simulink model "generic_IVS"  (R2024a)
settings: Solver=FixedStepDiscrete  StartTime=0.0  StopTime=inf  FixedStep=0.001  RelTol=1e-3  EnableMultiTasking=on
undefined symbols (not defined in the file): filtered_route_waypoint_raw, route1_waypoint_x, route1_waypoint_y, route2_waypoint_raw, route2_waypoint_x, route2_waypoint_y, route3_waypoint_x, route3_waypoint_y, route4_waypoint_x, route4_waypoint_y, route5_waypoint_x, route5_waypoint_y
libraries: CarMaker4SL x125, slpidlib x7, simulink x1, robotalgslib x1
(part 5 of 5)

== matlab function generic_IVS/CarMaker/Subsystem/Final Project/Scenario 1/Triggered Subsystem2/Function-Call Subsystem/MATLAB Function4 ==
  data: start input; goal input; obstacle_list input; full_path output
function full_path = main_rrt_rs(start, goal, obstacle_list) %#codegen
    disp("MAP making start")
    space = [5.5, 47.5, -44.9, -4.1];
    max_iter = 15000; step_size = 0.4; goal_sample_rate = 0.6; radius = 15;
    MAX_NODES = 5000;
    default_node = struct('pos', zeros(1,3), 'parent', int32(0), 'cost', Inf);
    nodes = repmat(default_node, 1, MAX_NODES);
    nodes(1).pos = start(:)';
    nodes(1).parent = int32(0);
    nodes(1).cost = 0.0;
    node_count = int32(1);
    goal = reshape(goal, 1, 3);
    start = reshape(start, 1, 3);

    c_best = inf; best_goal_node = int32(-1);

    for iter = 1:max_iter
        if rand < goal_sample_rate
            sample = goal;
        elseif isfinite(c_best)
            sample = informed_sample(start, goal, c_best, space);
        else
            sample = [ ...
                rand_range(space(1), space(2)), ...
                rand_range(space(3), space(4)), ...
                rand * 2 * pi ...
                ];
        end
        sample = reshape(sample, 1, 3);
        min_dist = inf;
        nearest_id = int32(1);
        for i = 1:node_count
            d = norm(nodes(i).pos(1:2) - sample(1:2));
            if d < min_dist
                min_dist = d;
                nearest_id = int32(i);
            end
        end
        nearest_node = nodes(nearest_id);

        theta = atan2(sample(2) - nearest_node.pos(2), sample(1) - nearest_node.pos(1));
        new_pos = [nearest_node.pos(1:2) + step_size * [cos(theta), sin(theta)], theta];

        if ~collision_check_line(nearest_node.pos, new_pos, obstacle_list, space)
            new_node = struct('pos', new_pos, ...
                'parent', int32(nearest_id), ...
                'cost', nearest_node.cost + norm(new_pos(1:2) - nearest_node.pos(1:2)));

            for i = 1:node_count
                if norm(nodes(i).pos(1:2) - new_node.pos(1:2)) < radius
                    temp_cost = nodes(i).cost + norm(nodes(i).pos(1:2) - new_node.pos(1:2));
                    if temp_cost < new_node.cost && ~collision_check_line(nodes(i).pos, new_node.pos, obstacle_list, space)
                        new_node.cost = temp_cost;
                        new_node.parent = int32(i);
                    end
                end
            end

            if node_count < MAX_NODES
                node_count = node_count + 1;
                nodes(node_count) = new_node;
            end

            if norm(new_node.pos(1:2) - goal(1:2)) < 10 && abs(wrapToPi(new_node.pos(3) - goal(3))) < deg2rad(360)
                if new_node.cost < c_best
                    c_best = new_node.cost;
                    best_goal_node = node_count;
                end
            end
        end
    end

    function yaw = wrapToPi(yaw)
        while yaw > pi
            yaw = yaw - 2*pi;
        end
        while yaw < -pi
            yaw = yaw + 2*pi;
        end
    end

    if best_goal_node > 0
        path_temp = zeros(300, 3);
        count = int32(0);
        current = best_goal_node;
        while current > 0
            count = count + 1;
            path_temp(count,:) = nodes(current).pos;
            current = nodes(current).parent;
        end
        rrt_path = flipud(path_temp(1:count,:));
        rrt_path = path_clothoid_smoothing(rrt_path);
        n_rrt = size(rrt_path, 1);

        full_path = NaN(300,3);
        full_path(1:n_rrt, :) = rrt_path;
        full_path(n_rrt + 1, :) = goal;  % ✅ goal을 마지막에 추가
    else
        full_path = NaN(300,3);
        disp('No Map Path!')
    end

    function r = rand_range(a, b) %#codegen
        r = a + (b - a) * rand;
    end

    disp("MAP function finish")
end
function sample = informed_sample(start, goal, c_max, space) %#codegen
    % === 고정된 출력: 반드시 [1×3] 벡터 ===
    sample = zeros(1, 3);

    % === 타원 파라미터 계산 ===
    c_min = norm(goal(1:2) - start(1:2));
    a = c_max / 2;
    b = sqrt(max(1e-6, c_max^2 - c_min^2)) / 2;
    theta = atan2(goal(2) - start(2), goal(1) - start(1));
    cos_t = cos(theta);
    sin_t = sin(theta);
    mid = 0.5 * (start(1:2) + goal(1:2));

    % === 고정 반복 횟수 시도 (예: 50회) ===
    for i = 1:50
        x = a * (2 * rand - 1);  % [-a, a]
        y = b * (2 * rand - 1);  % [-b, b]

        % 타원 내부 점만 사용
        if (x^2 / a^2 + y^2 / b^2) <= 1
            pos_x = cos_t * x - sin_t * y + mid(1);
            pos_y = sin_t * x + cos_t * y + mid(2);
            yaw   = 2 * pi * rand;

            sample(1) = pos_x;
            sample(2) = pos_y;
            sample(3) = yaw;
            return;
        end
    end

    % 실패 시 fallback: goal 반환
    sample = goal(:)';  % [1×3] 형태 유지
end

function smooth_path = path_clothoid_smoothing(path)
    if size(path, 1) < 3
        smooth_path = path;
        return;
    end

    fixed_points = false(size(path, 1), 1);
    for i = 2:size(path, 1) - 1
        prev = path(i - 1, 1:2);
        curr = path(i, 1:2);
        next = path(i + 1, 1:2);
        angle1 = atan2(curr(2) - prev(2), curr(1) - prev(1));
        angle2 = atan2(next(2) - curr(2), next(1) - curr(1));
        if abs(angle1 - angle2) < deg2rad(5)
            fixed_points(i) = true;
        end
    end

    x = path(:, 1); y = path(:, 2); yaw = path(:, 3);
    s = cumsum([0; sqrt(diff(x).^2 + diff(y).^2)]);
    ts = linspace(0, s(end), 5 * numel(s));
    x_smooth = interp1(s(~fixed_points), x(~fixed_points), ts, 'pchip', 'extrap');
    y_smooth = interp1(s(~fixed_points), y(~fixed_points), ts, 'pchip', 'extrap');
    yaw_unwrap = unwrap(yaw);
    yaw_smooth = interp1(s(~fixed_points), yaw_unwrap(~fixed_points), ts, 'pchip', 'extrap');

    dx = gradient(x_smooth); dy = gradient(y_smooth);
    ddx = gradient(dx); ddy = gradient(dy);
    curvature = abs((dx .* ddy - dy .* ddx) ./ (dx.^2 + dy.^2).^(3/2));
    max_curvature = 0.05;

    for k = 2:length(curvature)
        if curvature(k) > max_curvature
            factor = max_curvature / curvature(k);
            x_smooth(k) = x_smooth(k-1) + factor * (x_smooth(k) - x_smooth(k-1));
            y_smooth(k) = y_smooth(k-1) + factor * (y_smooth(k) - y_smooth(k-1));
        end
    end
    smooth_path = [x_smooth',...
                    y_smooth',...
                    wrapToPi(yaw_smooth')];
end





function is_collision = collision_check_line(start_pos, end_pos, obstacle_list, space) %#codegen
    % 간단한 선분-장애물 교차 검사: 샘플링 방식 사용
    n = 10;
    is_collision = false;
    for i = 0:n
        t = i / n;
        pos = (1 - t) * start_pos + t * end_pos;
        if collision_check_point(pos, obstacle_list, space)
            is_collision = true;
            return;
        end
    end
end

function is_collision = collision_check_point(pos, obstacle_list, space)
    x = pos(1); y = pos(2);
    if x < space(1) || x > space(2) || y < space(3) || y > space(4)
        is_collision = true;
        return;
    end
    is_collision = false;
    for i = 1:size(obstacle_list, 1)
        dx = x - obstacle_list(i,1);
        dy = y - obstacle_list(i,2);
        if hypot(dx, dy) < obstacle_list(i,3) + 1.5
            is_collision = true;
            return;
        end
    end
end

== matlab function generic_IVS/CarMaker/Subsystem/Final Project/Scenario 1/Tollgate/Get frenet1/MATLAB Function2 ==
  settings: sampleTime=0.05
  data: x input; y input; mapx input; mapy input; next_wp input; frenet_s output; frenet_d output; n_x output; n_y output
function [frenet_s, frenet_d,n_x, n_y] = get_frenet(x, y, mapx, mapy, next_wp)

% 예외 처리: 첫 번째 웨이포인트면 1로 고정
if next_wp == 1
    prev_wp = 1;
else
    prev_wp = next_wp - 1;
end

% 웨이포인트 벡터 (경로 벡터)
n_x = mapx(next_wp) - mapx(prev_wp);
n_y = mapy(next_wp) - mapy(prev_wp);
x_x = x - mapx(prev_wp);
x_y = y - mapy(prev_wp);

% 투영 계산 (단위가 아닌 비율)
proj_norm = (x_x * n_x + x_y * n_y) / (n_x^2 + n_y^2);
proj_x = proj_norm * n_x;
proj_y = proj_norm * n_y;

% Frenet d 계산 (측방 오차)
frenet_d = sqrt((x_x - proj_x)^2 + (x_y - proj_y)^2);

% 외적 계산 (왼쪽/오른쪽 판단)
ego_vec = [x - mapx(prev_wp); y - mapy(prev_wp); 0];
map_vec = [n_x; n_y; 0];
d_cross = cross(ego_vec, map_vec);

if d_cross(3) > 0
    frenet_d = -frenet_d;
end

% Frenet s 계산 (누적 거리)
frenet_s = 0;
for i = 1:(prev_wp - 1)
    dx = mapx(i+1) - mapx(i);
    dy = mapy(i+1) - mapy(i);
    frenet_s = frenet_s + sqrt(dx^2 + dy^2);
end

frenet_s = frenet_s + sqrt(proj_x^2 + proj_y^2);

== matlab function generic_IVS/CarMaker/Subsystem/Final Project/Scenario 1/Tollgate/Get frenet1/MATLAB Function3 ==
  data: route2_waypoint_raw input; map_x output; map_y output
function [map_x,map_y] = map(route2_waypoint_raw)

map_x = route2_waypoint_raw(:,1);
map_y = route2_waypoint_raw(:,2);

== matlab function generic_IVS/CarMaker/Subsystem/Final Project/Scenario 1/Tollgate/Get frenet1/MATLAB Function4 ==
  data: frenet_s_in input; frenet_s_out output
function frenet_s_out = safe_frenet_s(frenet_s_in)
% 입력:
%   s_in  : 현재 계산된 frenet_s
% 출력:
%   s_out : 점프가 제한된 frenet_s 출력

    % 이전 frenet_s 저장용 persistent 변수
    persistent prev_s
    if isempty(prev_s)
        prev_s = 0;
    end

    % 허용 가능한 최대 변화량 (단위: m)
    THRESHOLD = 900.0;

    % 변화량이 너무 크면 이전 값 유지
    if abs(frenet_s_in - prev_s) > THRESHOLD
        frenet_s_out = prev_s;
    else
        frenet_s_out = frenet_s_in;
        prev_s = frenet_s_in;
    end
end

== matlab function generic_IVS/CarMaker/Subsystem/Final Project/Scenario 1/Tollgate/ACC PD1 ==
  settings: sampleTime=0.05
  data: obs_s_array input; desired_ax output; ego_s input; error_min output; desired_ax_cruise input; ego_d input; d_array input
function [desired_ax, error_min] = longitudinal_space_pid_controller_traffic(obs_s_array, ego_s, desired_ax_cruise, ego_d, d_array)
% obs_s_array : 8×1 double (각 traffic 차량의 s 좌표)
% ego_s       : 자차량 s 좌표
% desired_ax  : 가속도 출력 (m/s^2)
% error_min   : 선택된 전방 차량과의 거리 오차
% ego_d       : 자차의 d 좌표 (자차와 각 traffic의 d 값 차이 비교)
% d_array     : 각 traffic 차량들의 d 좌표

    % === PID gain 설정 ===
    Kp = 0.17; %0.4, 0.2, 0.3
    Ki = 0;
    Kd = 0;

    % === 목표 간격 ===
    target_distance = 29;  %m
    % 30, 25, 30, 28

    % === 상태 유지용 변수 ===
    persistent integral_error prev_error
    if isempty(integral_error)
        integral_error = 0;
        prev_error = 0;
    end

    dt = 0.05;  % 샘플링 주기

    % === 전방 차량 필터링 ===
    delta_s = obs_s_array - ego_s;
    front_idx = find(delta_s > 0);

    if isempty(front_idx)
        % 전방 차량 없음 → 정상 주행 유지 (가속)
        desired_ax = desired_ax_cruise;
        error_min = NaN;
        return;
    end

    % === 가장 가까운 전방 차량 선택 및 d 차이 확인 ===
    target_idx = -1;
    for i = 1:length(front_idx)
        idx = front_idx(i);
        d_diff = abs(ego_d - d_array(idx)); % 자차와 각 traffic 차량 간의 d 차이

        if d_diff < 1.75
            target_idx = idx;
            break;  % d 차이가 1.75보다 작으면 해당 차량을 선택
        end
    end

    % d 차이가 1.75보다 작은 차량이 없다면 크루즈 유지
    if target_idx == -1
        desired_ax = desired_ax_cruise;
        error_min = NaN;
        return;
    end

    % === 선택된 차량의 s 값으로 거리 계산 ===
    min_dist = delta_s(target_idx);
    % error_min 계산: 선택된 전방 차량과 자차 간의 거리 차이
    error_min = min_dist - target_distance;

    % === PID 계산 ===
    integral_error = integral_error + error_min * dt;
    derivative_error = (error_min - prev_error) / dt;

    % === s 거리 계산 후 ACC 작동 여부 ===
    if min_dist > target_distance
        % 전방 차량과의 거리가 목표 거리보다 크면 cruise 유지
        desired_ax = desired_ax_cruise;
    else
        % 그렇지 않으면 PID로 가속도 조절
        desired_ax = Kp * error_min + Ki * integral_error + Kd * derivative_error;
    end

    % === 상태 업데이트 ===
    prev_error = error_min;
end

%%
% function [desired_ax, error_min] = longitudinal_space_pid_controller_traffic(obs_s_array, ego_s, desired_ax_cruise, ego_d, d_array)
% % obs_s_array : 8×1 double (각 traffic 차량의 s 좌표)
% % ego_s       : 자차량 s 좌표
% % desired_ax  : 가속도 출력 (m/s^2)
% % error_min   : 선택된 전방 차량과의 거리 오차
% % ego_d       : 자차의 d 좌표 (자차와 각 traffic의 d 값 차이 비교)
% % d_array     : 각 traffic 차량들의 d 좌표
% 
%     % === PID gain 설정 ===
%     Kp = 1.2;%1.6;
%     Ki = 0.1;%0.1;
%     Kd = 0.038;%0.3;
% 
%     % === 목표 간격 ===
%     target_distance = 20;  % m
% 
%     % === 상태 유지용 변수 ===
%     persistent integral_error prev_error
%     if isempty(integral_error)
%         integral_error = 0;
%         prev_error = 0;
%     end
% 
%     dt = 0.001;  % 샘플링 주기
% 
%     % === 전방 차량 필터링 ===
%     delta_s = obs_s_array - ego_s;
%     front_idx = find(delta_s > 0);
% 
%     if isempty(front_idx)
%         % 전방 차량 없음 → 정상 주행 유지 (가속)
%         desired_ax = desired_ax_cruise;
%         error_min = NaN;
%         return;
%     end
% 
%     % === 가장 가까운 전방 차량 선택 및 d 차이 확인 ===
%     target_idx = -1;
%     for i = 1:length(front_idx)
%         idx = front_idx(i);
%         d_diff = abs(ego_d - d_array(idx)); % 자차와 각 traffic 차량 간의 d 차이
% 
%         if d_diff < 1.75
%             target_idx = idx;
%             break;  % d 차이가 1.75보다 작으면 해당 차량을 선택
%         end
%     end
% 
%     % d 차이가 1.75보다 작은 차량이 없다면 크루즈 유지
%     if target_idx == -1
%         desired_ax = desired_ax_cruise;
%         error_min = NaN;
%         return;
%     end
% 
%     % === 선택된 차량의 s 값으로 거리 계산 ===
%     min_dist = delta_s(target_idx);
%     % error_min 계산: 선택된 전방 차량과 자차 간의 거리 차이
%     error_min = min_dist - target_distance;
% 
%     % === PID 계산 ===
%     integral_error = integral_error + error_min * dt;
%     derivative_error = (error_min - prev_error) / dt;
% 
%     % === s 거리 계산 후 ACC 작동 여부 ===
%     if min_dist > target_distance +30
%         % 전방 차량과의 거리가 목표 거리보다 크면 cruise 유지
%         desired_ax = desired_ax_cruise;
%     else
%         % 그렇지 않으면 PID로 가속도 조절
%         desired_ax = Kp * error_min + Ki * integral_error + Kd * derivative_error;
%     end
% 
%     % === 상태 업데이트 ===
%     prev_error = error_min;
% end

== matlab function generic_IVS/CarMaker/Subsystem/Final Project/Scenario 1/Drive/MATLAB Function1 ==
  settings: sampleTime=0.1
  data: x input; x_best output; y input; v input; map_x input; map_y input; obs_x input; obs_y input; y_best output; x_all output; y_all output; obs_Vx input; obs_Vy input; obs_ax input; obs_ay input; predicted_traj_x output; predicted_traj_y output; front_obstacle_flag output; road_curvature output

function [x_best, y_best, x_all, y_all, predicted_traj_x, predicted_traj_y, front_obstacle_flag, road_curvature] = ...
    FrenetTrajectoryGenerator(x, y, v, map_x, map_y, ...
    obs_x, obs_y, obs_Vx, obs_Vy, obs_ax, obs_ay)

% === 설정 ===
DF_set = [-3.5, 0, 3.5];  
K_J = 0.1; K_T = 0.1; K_D = 10.0; K_V = 1.0;
K_LAT = 2.0; K_LON = 1.0; K_SAFE_DIST = 100.0;

target_speed = 15;
T = 1.2; dt = 0.05;
ego_radius = 1.5;
LANE_WIDTH = 3.5;

M = length(DF_set);
N = round(T / dt);

x_all = zeros(N, M);
y_all = zeros(N, M);

obs_r = 2.0;
num_obs = length(obs_x);

% === 기준 경로 길이 계산 ===
map_s = zeros(length(map_x), 1);
for i = 2:length(map_x)
    dx = map_x(i) - map_x(i-1);
    dy = map_y(i) - map_y(i-1);
    map_s(i) = map_s(i-1) + hypot(dx, dy);
end

% === Ego 차량 위치 변환 ===
[s0, d0] = getFrenet(x, y, map_x, map_y, map_s);
si = s0; si_d = v; si_dd = 0;
di = d0; di_d = 0; di_dd = 0;

% === 주변 차량 Frenet 기반 예측 정보 ===
pred_vehicles = zeros(num_obs, 3);  % [s0, v0, a0]
pred_d0 = zeros(num_obs, 1);        % 초기 lateral offset
predicted_traj_x = zeros(N, num_obs);
predicted_traj_y = zeros(N, num_obs);

for j = 1:num_obs
    [s_obs, d_obs] = getFrenet(obs_x(j), obs_y(j), map_x, map_y, map_s);
    pred_d0(j) = d_obs;

    idx = find(map_s > s_obs,1)-1;
    idx = max(min(idx,length(map_x)-1),1);
    dx = map_x(idx+1)-map_x(idx);
    dy = map_y(idx+1)-map_y(idx);
    heading = atan2(dy,dx);

    vx = obs_Vx(j); vy = obs_Vy(j);
    ax = obs_ax(j); ay = obs_ay(j);

    v0 = vx*cos(heading) + vy*sin(heading);
    a0 = ax*cos(heading) + ay*sin(heading);

    pred_vehicles(j,:) = [s_obs, v0, a0];

    for i = 1:N
        t = (i-1)*dt;
        s_pred = s_obs + v0*t + 0.5*a0*t^2;
        d_pred = d_obs;
        [x_pred, y_pred] = getCartesian(s_pred, d_pred, map_x, map_y, map_s);
        predicted_traj_x(i,j) = x_pred;
        predicted_traj_y(i,j) = y_pred;
    end
end

% === Trajectory 후보 생성 및 평가 ===
costs = inf(1, M);
trajectories = cell(M,2);

for k = 1:M
    d_target = DF_set(k);

    % Lateral (Quintic)
    a0 = di; a1 = di_d; a2 = 0.5 * di_dd;
    A_lat = [T^3 T^4 T^5; 3*T^2 4*T^3 5*T^4; 6*T 12*T^2 20*T^3];
    b_lat = [d_target - a0 - a1*T - a2*T^2; -a1 - 2*a2*T; -2*a2];
    coeff_d = A_lat \ b_lat;

    % Longitudinal (Quartic)
    b0 = si; b1 = si_d; b2 = 0.5 * si_dd;
    A_lon = [3*T^2 4*T^3; 6*T 12*T^2];
    b_lon = [target_speed - b1 - 2*b2*T; -2*b2];
    coeff_s = A_lon \ b_lon;

    s_traj = zeros(N,1); d_traj = zeros(N,1);
    x_traj = zeros(N,1); y_traj = zeros(N,1);
    jerk_d = 0; jerk_s = 0;
    is_collision = false;
    min_gap = inf;

    for i = 1:N
        t = (i-1)*dt;
        s_t = b0 + b1*t + b2*t^2 + coeff_s(1)*t^3 + coeff_s(2)*t^4;
        d_t = a0 + a1*t + a2*t^2 + coeff_d(1)*t^3 + coeff_d(2)*t^4 + coeff_d(3)*t^5;

        s_traj(i) = s_t; d_traj(i) = d_t;

        j_d = 6*coeff_d(1) + 24*coeff_d(2)*t + 60*coeff_d(3)*t^2;
        j_s = 6*coeff_s(1) + 24*coeff_s(2)*t;
        jerk_d = jerk_d + j_d^2;
        jerk_s = jerk_s + j_s^2;

        [xg, yg] = getCartesian(s_t, d_t, map_x, map_y, map_s);
        x_traj(i) = xg;
        y_traj(i) = yg;

        % 정적 장애물: 같은 차선일 때만 판단
        for j = 1:num_obs
            [~, d_obs_static] = getFrenet(obs_x(j), obs_y(j), map_x, map_y, map_s);
            if abs(d_obs_static - d_t) < LANE_WIDTH / 2
                dist = hypot(xg - obs_x(j), yg - obs_y(j));
                if dist < (ego_radius + obs_r)
                    is_collision = true;
                end
            end
        end

        % 동적 장애물: 같은 차선만 판단
        for j = 1:num_obs
            s_pred = pred_vehicles(j,1) + pred_vehicles(j,2)*t + 0.5*pred_vehicles(j,3)*t^2;
            d_pred = pred_d0(j);
            ds = s_pred - s_t;
            dd = d_pred - d_t;
            dist_frenet = sqrt(ds^2 + dd^2);

            if abs(dd) < LANE_WIDTH / 2
                if dist_frenet < (ego_radius + obs_r)
                    is_collision = true;
                end
                if ds >= 0
                    min_gap = min(min_gap, ds);
                end
            end
        end
    end

    x_all(:,k) = x_traj;
    y_all(:,k) = y_traj;

    if ~is_collision
        d_diff = (d_traj(end))^2;
        v_diff = (target_speed - (s_traj(end)-s_traj(1))/T)^2;
        cost_lat = K_J*jerk_d + K_T*T + K_D*d_diff;
        cost_lon = K_J*jerk_s + K_T*T + K_V*v_diff;
        safe_cost = 0;
        if min_gap < 15
            safe_cost = K_SAFE_DIST * (15 - min_gap)^2;
        end
        costs(k) = K_LAT*cost_lat + K_LON*(cost_lon + safe_cost);
    end

    trajectories{k,1} = x_traj;
    trajectories{k,2} = y_traj;
end

% === 최적 trajectory 선택 ===
persistent prev_best_idx hold_count
if isempty(prev_best_idx)
    prev_best_idx = 2;
    hold_count = 0;
end

[best_cost, new_best_idx] = min(costs);
threshold = 5.0;
hold_limit = 3.0 / dt;
current_cost = costs(prev_best_idx);

if (new_best_idx ~= prev_best_idx) && ...
        (best_cost + threshold < current_cost || hold_count >= hold_limit)
    prev_best_idx = new_best_idx;
    hold_count = 0;
else
    new_best_idx = prev_best_idx;
    hold_count = hold_count + 1;
end

x_best = trajectories{new_best_idx,1};
y_best = trajectories{new_best_idx,2};

% === 전방 장애물 플래그 ===
front_obstacle_flag = 0;
SAFE_DETECT_DIST = 40;
for j = 1:num_obs
    s_pred = pred_vehicles(j,1);
    d_pred = pred_d0(j);
    ds = s_pred - s0;
    dd = d_pred - d0;
    if ds > 0 && ds < SAFE_DETECT_DIST && abs(dd) < LANE_WIDTH / 2
        front_obstacle_flag = 13;
        break;
    end
end

% === 전방 곡률 계산 ===
road_curvature = 0;
num_curv_pts = 10;
idx = find(map_s > s0, 1);
idx = idx(1);
if ~isempty(idx) && (idx + num_curv_pts <= length(map_s))
    xs = map_x(idx:idx+num_curv_pts);
    ys = map_y(idx:idx+num_curv_pts);
    dx = gradient(xs);
    dy = gradient(ys);
    ddx = gradient(dx);
    ddy = gradient(dy);
    kappa = abs(dx .* ddy - dy .* ddx) ./ (dx.^2 + dy.^2).^(3/2);
    kappa(~isfinite(kappa)) = 0;
    road_curvature = mean(kappa);
end

end



%% === 보조 함수 ===

function [s, d] = getFrenet(x, y, mapx, mapy, maps)
min_dist = inf; idx = 1;
for i = 1:length(mapx)-1
    dist = hypot(x - mapx(i), y - mapy(i));
    if dist < min_dist
        min_dist = dist;
        idx = i;
    end
end
dx = mapx(idx+1) - mapx(idx);
dy = mapy(idx+1) - mapy(idx);
seg_len = hypot(dx, dy);
proj = ((x - mapx(idx)) * dx + (y - mapy(idx)) * dy) / seg_len^2;
proj_x = mapx(idx) + proj * dx;
proj_y = mapy(idx) + proj * dy;
d = (x - proj_x) * (-dy/seg_len) + (y - proj_y) * (dx/seg_len);
s = maps(idx) + proj * seg_len;
end

function [x, y] = getCartesian(s, d, mapx, mapy, maps)
if s >= maps(end)
    s = maps(end) - 0.001;
end
idx_array = find(maps > s, 1);
if isempty(idx_array)
    idx = length(maps) - 1;
else
    idx = idx_array - 1;
end
if idx < 1
    idx = 1;
elseif idx >= length(mapx)
    idx = length(mapx) - 1;
end
mx0 = mapx(idx); mx1 = mapx(idx+1);
my0 = mapy(idx); my1 = mapy(idx+1);
dx_val = mx1 - mx0;
dy_val = my1 - my0;
heading = atan2(dy_val, dx_val);
ds = s - maps(idx);
base_x = mx0 + ds * cos(heading);
base_y = my0 + ds * sin(heading);
x = base_x - d * sin(heading);
y = base_y + d * cos(heading);
end

== matlab function generic_IVS/CarMaker/Subsystem/Final Project/Scenario 1/Drive/MATLAB Function4  ==
  settings: updateMethod=DISCRETE
  data: waypoint_x input; waypoint_y input; local_waypoints_ output; vehicle_position input; head input
function local_waypoints_ = global_to_local_waypoints(waypoint_x, waypoint_y, vehicle_position, head)

    % 초기화
    num_points = size(waypoint_x, 1);
    local_waypoints_ = NaN(num_points, 2);  % [x_local, y_local]

    % 차량 위치 추출
    ego_x = vehicle_position(1);
    ego_y = vehicle_position(2);
    ego_yaw = head;

    % 회전 행렬 생성 (글로벌→로컬 변환)
    R = [cos(-ego_yaw) -sin(-ego_yaw); 
         sin(-ego_yaw)  cos(-ego_yaw)];

    count = 0;
    % 각 웨이포인트에 대해 변환 수행
    for i = 1:num_points
        % 글로벌 좌표에서 차량까지의 상대 위치
        dx = waypoint_x(i) - ego_x;  % X 좌표 차이
        dy = waypoint_y(i) - ego_y;  % Y 좌표 차이

        % 회전 변환 적용
        local_pos = R * [dx; dy];
        distance = sqrt(dx.^2 + dy.^2); % 차량으로부터 waypoint까지의 길이 계산

        % 시작 좌표 저장
        if count == 0 && local_pos(1) > 0 && distance < 15
            count = count + 1;
            local_waypoints_(count, :) = [local_pos(1) local_pos(2)];     % 로컬 x 좌표 
        end

        % 아래의 조건을 모두 만족하는 경우에만 좌표 저장
        % 1. x 좌표가 0보다 큰 경우
        % 2. x의 현재 좌표가 이전 x의 좌표보다 큰 경우
        % 3. 차량으로부터 waypoint까지의 길이가 30m 이내인 경우 (길이는 임의로 테스트 한 후 설정 가능할 듯)
        if count  ~= 0 && local_pos(1) > 0 && local_pos(1) > local_waypoints_(count, 1)  && distance < 15
            count = count + 1;
            local_waypoints_(count, :) = [local_pos(1) local_pos(2)];
        end
    end
end

== matlab function generic_IVS/CarMaker/Subsystem/Final Project/Scenario 1/PreParking/MATLAB Function4 ==
  settings: sampleTime=0.05
  data: poly_coeff input; lateral_error output; velocity input; lookahead_time input; x_lookahead output
function [lateral_error, x_lookahead] = compute_lateral_error(poly_coeff, velocity, lookahead_time)
    % Lookahead 지점 계산
    x_lookahead = velocity * lookahead_time + 2.9;

    % 경로 상의 lookahead 지점에서의 y값 계산
    y_desired = polyval(poly_coeff, x_lookahead);

    % lateral error : 차량 y=0 위치와 경로 y_desired의 차이
    lateral_error = y_desired;
end
